simulink model "sampleModel1405"  (R2023a)
settings: Solver=VariableStepAuto  StartTime=0.0  StopTime=10.0  RelTol=1e-3
libraries: hdlsllib x3, simulink x1
settings Model: Creator=user1  LastModifiedBy=user1

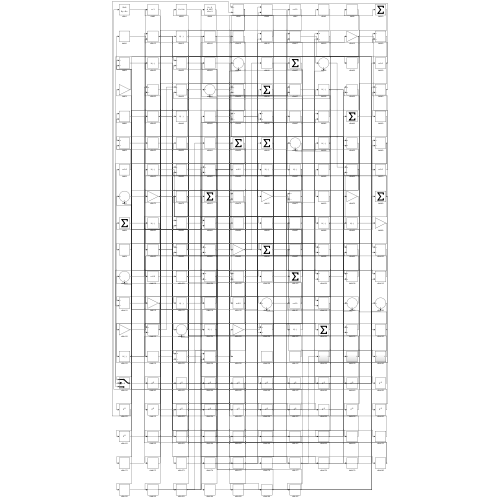
[thumbnail: Simulink's stored preview of the top-level diagram]
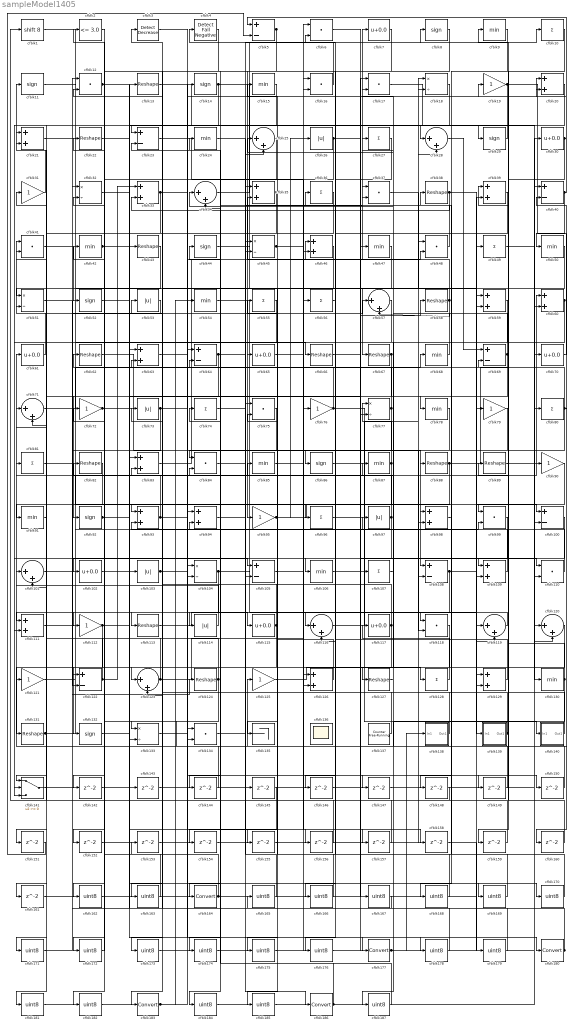
== system sampleModel1405 ==
  cfblk1 : ArithShift  BitShiftNumber=8
  cfblk{10,27,36,49,55..56,74,80..81,96,107,128} (12 alike) : Sum  Inputs=+
  cfblk{5,23,40,64,69,100,105,108,122} (9 alike) : Sum  Inputs=+-
  cfblk{25,28,34,57,71,101,116,119..120,123} (10 alike) : Sum  Inputs=|++
  cfblk{7,30,61,65,70,102,115,117} (8 alike) : Bias  Bias=0.0  SaturateOnIntegerOverflow=off
  cfblk{26,53,73,97,103,114} (6 alike) : Abs  SaturateOnIntegerOverflow=off
  cfblk{18,32,45,51,77,104,133} (7 alike) : Product  Inputs=*/  RndMeth=Zero  SaturateOnIntegerOverflow=on
  cfblk{9,15,24,42,47,50,54,68,78,85,87,91,106,130} (14 alike) : MinMax
  cfblk{20..21,33,35,39,46,59..60,63,83,93..94,98,109,111,126,129} (17 alike) : Sum
  cfblk{8,11,14,29,44,52,86,92,132} (9 alike) : Signum
  cfblk{6,12,16..17,37,41,48,75,84,99,110,118,134} (13 alike) : DotProduct  OutDataTypeStr=Inherit: Inherit via internal rule
  cfblk{19,31,72,76,79,90,95,112,121,125} (10 alike) : Gain
  cfblk{13,22,38,43,58,62,66..67,82,88..89,113,124,127,131} (15 alike) : Reshape
  cfblk135 : Terminator
  cfblk136 : Scope
      settings: Floating=on
  cfblk137 : hdlsllib/Sources/Counter Free-Running  NumBits=16  tsamp=-1
  cfblk138 : Subsystem
      settings: LibrarySourceBlock=|
      | hdlsllib/Ports &
      | Subsystems/Subsystem
  cfblk139 : Subsystem
      settings: LibrarySourceBlock=|
      | hdlsllib/Ports &
      | Subsystems/Subsystem
  cfblk140 : Subsystem
      settings: LibrarySourceBlock=|
      | hdlsllib/Ports &
      | Subsystems/Subsystem
  cfblk141 : Switch  SaturateOnIntegerOverflow=off  InputSameDT=off
  cfblk{142..161} (20 alike) : Delay  SampleTime=1
  cfblk{162..163,165..176,178..179,181..182,184..185,187} (21 alike) : DataTypeConversion  OutDataTypeStr=uint8  SaturateOnIntegerOverflow=off  RndMeth=Floor
  cfblk{164,177,180,183,186} (5 alike) : DataTypeConversion  SaturateOnIntegerOverflow=off  RndMeth=Floor
  cfblk2 : hdlsllib/Logic and Bit Operations/Compare To Constant  relop=<=  const=3.0  OutDataTypeStr=boolean
  cfblk3 : simulink/Logic and Bit Operations/Detect Decrease  vinit=0.0  OutDataTypeStr=boolean
      settings: LibrarySourceBlock=|
      | hdlsllib/Logic and Bit
      | Operations/Detect
      | Decrease
  cfblk4 : hdlsllib/Logic and Bit Operations/Detect Fall Negative  vinit=0  OutDataTypeStr=boolean
  wires:
  cfblk87/1 -> cfblk77/1, cfblk182/1
  cfblk83/1 -> cfblk7/1
  cfblk18/1 -> cfblk28/1
  cfblk131/1 -> cfblk60/1, cfblk124/1
  cfblk67/1 -> cfblk92/1, cfblk114/1
  cfblk54/1 -> cfblk116/1
  cfblk1/1 -> cfblk66/1
  cfblk28/1 -> cfblk69/1
  cfblk88/1 -> cfblk39/1, cfblk141/1
  cfblk8/1 -> cfblk95/1
  cfblk50/1 -> cfblk67/1
  cfblk130/1 -> cfblk89/1, cfblk187/1
  cfblk126/1 -> cfblk55/1
  cfblk14/1 -> cfblk76/1, cfblk133/1
  cfblk9/1 -> cfblk78/1
  cfblk73/1 -> cfblk94/1, cfblk122/2
  cfblk109/1 -> cfblk46/1
  cfblk111/1 -> cfblk48/1
  cfblk71/1 -> cfblk68/1
  cfblk38/1 -> cfblk139/1(In1), cfblk110/1, cfblk33/2
  cfblk42/1 -> cfblk43/1, cfblk98/2
  cfblk76/1 -> cfblk140/1(In1), cfblk15/1
  cfblk68/1 -> cfblk34/1
  cfblk19/1 -> cfblk125/1, cfblk141/3, cfblk168/1
  cfblk34/1 -> cfblk8/1
  cfblk29/1 -> cfblk23/1
  cfblk113/1 -> cfblk115/1
  cfblk95/1 -> cfblk100/1, cfblk26/1
  cfblk49/1 -> cfblk100/2
  cfblk125/1 -> cfblk128/1
  cfblk40/1 -> cfblk50/1, cfblk20/2
  cfblk23/1 -> cfblk46/2
  cfblk72/1 -> cfblk126/1, cfblk118/2
  cfblk17/1 -> cfblk70/1
  cfblk124/1 -> cfblk61/1, cfblk72/1, cfblk172/1
  cfblk16/1 -> cfblk4/1
  cfblk74/1 -> cfblk186/1
  cfblk112/1 -> cfblk131/1, cfblk99/2
  cfblk59/1 -> cfblk91/1
  cfblk44/1 -> cfblk129/1
  cfblk57/1 -> cfblk65/1
  cfblk63/1 -> cfblk177/1
  cfblk92/1 -> cfblk13/1, cfblk169/1
  cfblk121/1 -> cfblk17/1
  cfblk118/1 -> cfblk132/1
  cfblk61/1 -> cfblk41/1
  cfblk26/1 -> cfblk113/1, cfblk108/2
  cfblk117/1 -> cfblk36/1, cfblk64/2, cfblk166/1
  cfblk114/1 -> cfblk101/1
  cfblk140/1(Out1) -> cfblk9/1
  cfblk116/1 -> cfblk18/1
  cfblk15/1 -> cfblk101/2
  cfblk13/1 -> cfblk130/1
  cfblk21/1 -> cfblk93/1
  cfblk33/1 -> cfblk14/1, cfblk151/1, cfblk152/1
  cfblk128/1 -> cfblk117/1
  cfblk31/1 -> cfblk11/1
  cfblk25/1 -> cfblk102/1
  cfblk62/1 -> cfblk108/1
  cfblk60/1 -> cfblk127/1, cfblk105/2
  cfblk43/1 -> cfblk51/1
  cfblk41/1 -> cfblk52/1
  cfblk5/1 -> cfblk84/1, cfblk122/1
  cfblk141/1 -> cfblk90/1
  cfblk89/1 -> cfblk30/1
  cfblk104/1 -> cfblk126/2, cfblk121/1
  cfblk37/1 -> cfblk59/2
  cfblk77/1 -> cfblk34/2, cfblk185/1
  cfblk12/1 -> cfblk29/1, cfblk77/2
  cfblk97/1 -> cfblk21/1, cfblk21/2, cfblk141/2
  cfblk119/1 -> cfblk112/1
  cfblk86/1 -> cfblk98/1
  cfblk75/1 -> cfblk164/1
  cfblk137/1 -> cfblk82/1
  cfblk101/1 -> cfblk57/1
  cfblk64/1 -> cfblk104/2, cfblk88/1, cfblk37/1, cfblk133/2, cfblk37/2
  cfblk96/1 -> cfblk109/1
  cfblk66/1 -> cfblk58/1
  cfblk106/1 -> cfblk107/1
  cfblk110/1 -> cfblk53/1
  cfblk58/1 -> cfblk35/2, cfblk57/2
  cfblk70/1 -> cfblk40/2
  cfblk138/1(Out1) -> cfblk83/2
  cfblk51/1 -> cfblk105/1
  cfblk120/1 -> cfblk183/1
  cfblk115/1 -> cfblk3/1, cfblk123/1
  cfblk80/1 -> cfblk62/1, cfblk42/1, cfblk160/1, cfblk174/1
  cfblk11/1 -> cfblk129/2
  cfblk45/1 -> cfblk20/1, cfblk119/2
  cfblk99/1 -> cfblk111/1
  cfblk134/1 -> cfblk180/1
  cfblk90/1 -> cfblk109/2
  cfblk53/1 -> cfblk51/2
  cfblk30/1 -> cfblk5/1, cfblk99/1
  cfblk91/1 -> cfblk71/2
  cfblk81/1 -> cfblk84/2
  cfblk105/1 -> cfblk56/1
  cfblk122/1 -> cfblk81/1, cfblk33/1
  cfblk48/1 -> cfblk23/2
  cfblk108/1 -> cfblk49/1, cfblk123/2
  cfblk123/1 -> cfblk22/1, cfblk97/1, cfblk41/2
  cfblk94/1 -> cfblk10/1
  cfblk139/1(Out1) -> cfblk44/1, cfblk12/2
  cfblk103/1 -> cfblk19/1, cfblk73/1
  cfblk78/1 -> cfblk86/1
  cfblk46/1 -> cfblk135/1
  cfblk39/1 -> cfblk96/1
  cfblk35/1 -> cfblk45/2, cfblk181/1
  cfblk107/1 -> cfblk27/1
  cfblk56/1 -> cfblk106/1
  cfblk69/1 -> cfblk118/1, cfblk25/1, cfblk161/1
  cfblk129/1 -> cfblk85/1
  cfblk127/1 -> cfblk87/1
  cfblk93/1 -> cfblk48/2, cfblk31/1
  cfblk55/1 -> cfblk111/2
  cfblk20/1 -> cfblk142/1
  cfblk142/1 -> cfblk35/1
  cfblk132/1 -> cfblk143/1
  cfblk143/1 -> cfblk18/2
  cfblk36/1 -> cfblk144/1
  cfblk144/1 -> cfblk83/1
  cfblk24/1 -> cfblk145/1
  cfblk27/1 -> cfblk146/1
  cfblk146/1 -> cfblk40/1
  cfblk84/1 -> cfblk147/1
  cfblk147/1 -> cfblk60/2
  cfblk98/1 -> cfblk148/1
  cfblk148/1 -> cfblk1/1
  cfblk65/1 -> cfblk149/1
  cfblk149/1 -> cfblk17/2
  cfblk133/1 -> cfblk150/1
  cfblk150/1 -> cfblk104/1
  cfblk151/1 -> cfblk5/2
  cfblk152/1 -> cfblk25/2
  cfblk153/1 -> cfblk28/2
  cfblk100/1 -> cfblk154/1
  cfblk154/1 -> cfblk45/1
  cfblk3/1 -> cfblk155/1
  cfblk155/1 -> cfblk59/1
  cfblk22/1 -> cfblk156/1
  cfblk156/1 -> cfblk71/1
  cfblk85/1 -> cfblk157/1
  cfblk157/1 -> cfblk93/2
  cfblk52/1 -> cfblk158/1
  cfblk10/1 -> cfblk159/1
  cfblk159/1 -> cfblk116/2
  cfblk160/1 -> cfblk69/2
  cfblk161/1 -> cfblk119/1
  cfblk2/1 -> cfblk162/1
  cfblk162/1 -> cfblk103/1
  cfblk4/1 -> cfblk163/1
  cfblk163/1 -> cfblk2/1
  cfblk164/1 -> cfblk153/1, cfblk39/2
  cfblk165/1 -> cfblk75/1
  cfblk166/1 -> cfblk75/2
  cfblk6/1 -> cfblk167/1
  cfblk167/1 -> cfblk165/1
  cfblk168/1 -> cfblk6/1
  cfblk169/1 -> cfblk6/2
  cfblk32/1 -> cfblk170/1
  cfblk170/1 -> cfblk38/1
  cfblk82/1 -> cfblk171/1
  cfblk171/1 -> cfblk32/1
  cfblk172/1 -> cfblk32/2
  cfblk47/1 -> cfblk173/1
  cfblk173/1 -> cfblk16/1
  cfblk174/1 -> cfblk47/1
  cfblk79/1 -> cfblk175/1
  cfblk175/1 -> cfblk16/2
  cfblk7/1 -> cfblk176/1
  cfblk176/1 -> cfblk79/1
  cfblk177/1 -> cfblk80/1, cfblk138/1(In1)
  cfblk102/1 -> cfblk178/1
  cfblk178/1 -> cfblk63/1
  cfblk158/1 -> cfblk179/1
  cfblk179/1 -> cfblk63/2
  cfblk180/1 -> cfblk12/1, cfblk94/2
  cfblk181/1 -> cfblk134/1
  cfblk182/1 -> cfblk134/2
  cfblk183/1 -> cfblk64/1, cfblk54/1
  cfblk145/1 -> cfblk184/1
  cfblk184/1 -> cfblk120/1
  cfblk185/1 -> cfblk120/2
  cfblk186/1 -> cfblk110/2, cfblk24/1
  cfblk187/1 -> cfblk74/1

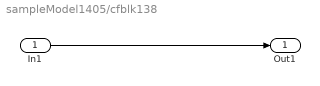
== system sampleModel1405/cfblk138 ==
  In1 : Inport
  Out1 : Outport
  wires:
  In1/1 -> Out1/1

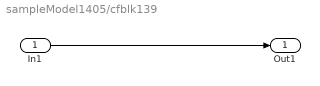
== system sampleModel1405/cfblk139 ==
  In1 : Inport
  Out1 : Outport
  wires:
  In1/1 -> Out1/1

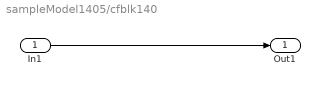
== system sampleModel1405/cfblk140 ==
  In1 : Inport
  Out1 : Outport
  wires:
  In1/1 -> Out1/1
